simulink model "Simscape_Simulink_Mass_Spring_Damper_RL"  (R2024b)
settings: Solver=VariableStepAuto  StartTime=0.0  StopTime=10.0  RelTol=1e-3
undefined symbols (not defined in the file or in its folder): DiscIntNeverNeededParam, X, Y, Z
libraries: sm_lib x10, nesl_utility x3, simulink x1, rllib x1
settings Model: Creator=JEETKUMAR PATEL  LastModifiedBy=JEETKUMAR PATEL

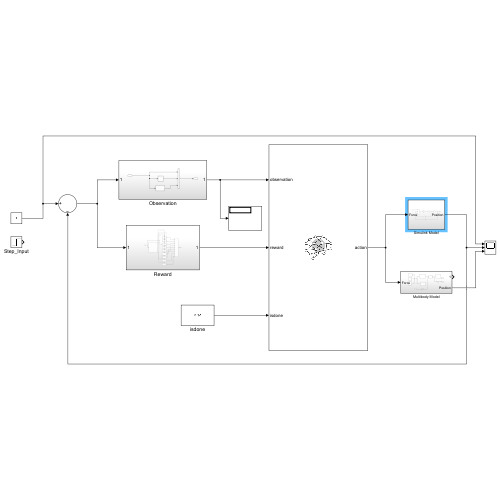
[thumbnail: Simulink's stored preview of the top-level diagram]
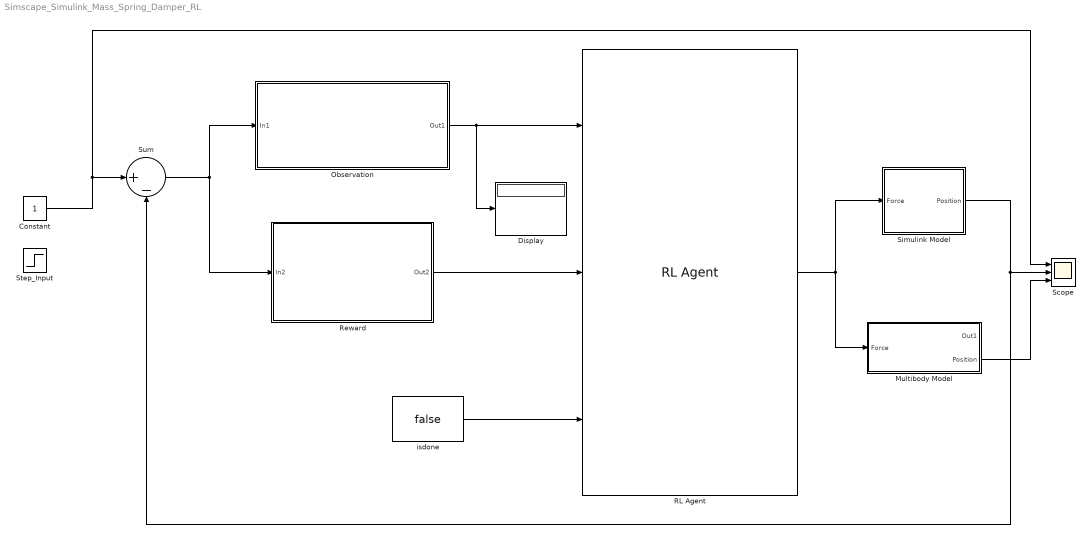
== system Simscape_Simulink_Mass_Spring_Damper_RL ==
  Constant : Constant
  Display : Display
  Multibody Model : Subsystem
  Observation : Subsystem
  RL Agent : rllib/RL Agent  Agent=agent  ExternalActionAsInput=off  ProvideLastAction=off  ProvideCumRwd=off  TreatAsDirectFeedthrough=on  UseStrictObservationDataTypes=off
  Reward : Subsystem
  Scope : Scope  NumInputPorts=3
  Simulink Model : Subsystem
  Step_Input : Step  SampleTime=0
  Sum : Sum  Inputs=|+-
  isdone : Constant  Value=false
  wires:
  Observation/1(Out1) -> RL Agent/1, Display/1
  Sum/1 -> Observation/1(In1), Reward/1(In2)
  Reward/1(Out2) -> RL Agent/2
  Constant/1 -> Sum/1, Scope/1
  Simulink Model/1(Position) -> Sum/2, Scope/2
  RL Agent/1 -> Multibody Model/1(Force), Simulink Model/1(Force)
  isdone/1 -> RL Agent/3
  Multibody Model/2(Position) -> Scope/3

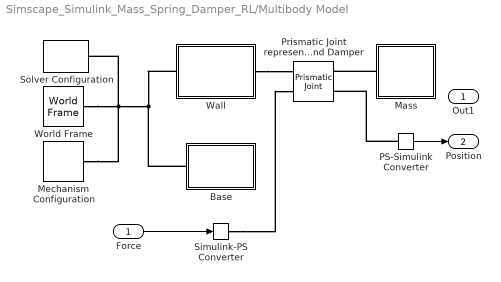
== system Simscape_Simulink_Mass_Spring_Damper_RL/Multibody Model ==
  Force : Inport
  Base : Subsystem
  Mass : Subsystem
  Mechanism Configuration : sm_lib/Utilities/Mechanism Configuration  UniformGravity=Constant  GravityVector=[0 0 -9.80665]  GravityVectorUnits=m/s^2  LinearizationDelta=0.001  JointModeTransitionNonlinearIterations=2
  PS-Simulink Converter : nesl_utility/PS-Simulink Converter  PhysicalDomain=network_engine_domain  SubClassName=ps_output  LeftPortType=input  RightPortType=output  PseudoPeriodic=off  Frequencies=[]  VectorFormat=1-D array  Unit=1  AffineConversion=off
  Prismatic Joint representing Spring and Damper : sm_lib/Joints/Prismatic Joint  JointMode=Normal  CompositeWrenchDir=FollowerOnBase  CompositeWrenchFrame=BaseFrame  SenseConstraintForce=off  SenseConstraintTorque=off  SenseTotalForce=off  SenseTotalTorque=off  PositionTargetSpecify=off  PositionTargetPriority=High  PositionTargetValue=0  PositionTargetValueUnits=m  VelocityTargetSpecify=off  VelocityTargetPriority=High  VelocityTargetValue=0  VelocityTargetValueUnits=m/s  EquilibriumPosition=0  EquilibriumPositionUnits=m  SpringStiffness=1  SpringStiffnessUnits=N/m  DampingCoefficient=1  DampingCoefficientUnits=N/(m/s)  LowerLimitSpecify=off  LowerLimitBound=-1  LowerLimitBoundUnits=m  LowerLimitStiffness=1e6  LowerLimitStiffnessUnits=N/m  LowerLimitDamping=1e3  LowerLimitDampingUnits=N/(m/s)  LowerLimitTransitionRegionWidth=1e-4  LowerLimitTransitionRegionWidthUnits=m  UpperLimitSpecify=off  UpperLimitBound=1  UpperLimitBoundUnits=m  UpperLimitStiffness=1e6  UpperLimitStiffnessUnits=N/m  UpperLimitDamping=1e3  UpperLimitDampingUnits=N/(m/s)  UpperLimitTransitionRegionWidth=1e-4  UpperLimitTransitionRegionWidthUnits=m  TorqueActuationMode=InputTorque  MotionActuationMode=ComputedMotion  SensePosition=on  SenseVelocity=off  SenseAcceleration=off  SenseTorqueForce=off  SenseLowerLimitTorqueForce=off  SenseUpperLimitTorqueForce=off
  Simulink-PS Converter : nesl_utility/Simulink-PS Converter  PhysicalDomain=network_engine_domain  SubClassName=ps_input  LeftPortType=input  RightPortType=output  PseudoPeriodic=off  Frequencies=[]  NoiseDistribution=none  NoiseParameters=[]  Unit=1  AffineConversion=off  FilteringAndDerivatives=provide  SimscapeFilterOrder=1  InputFilterTimeConstant=0.001  UdotUserProvided=0
  Solver Configuration : nesl_utility/Solver Configuration  PhysicalDomain=network_engine_domain  SubClassName=solver  LeftPortType=input  RightPortType=generic  Tones=[]  Harmonics=[]  SimulateNoise=off  Profile=off  UseLocalSampling=off  EnableSwitchedLinearOptims=on  FrequencyDomain=off  UseCCode=off  RelTol=0.001  AbsTol=1e-06  MinStep=1e-09  ToWorkspace=off  RevertToSquareIcSolve=off  NumHomotopyIterations=100  PhasorMode=off  PhasorModeNumHarmonics=1  ConsistencySolver=NEWTON_FTOL  IndexReductionMethod=DerivativeReplacement  DoDC=off  ResidualTolerance=1e-09  ConsistencyTolSource=GLOBAL  ConsistencyAbsTol=0.001  ConsistencyRelTol=0.001  ConsistencyTolFactor=0.001  UseLocalSolver=off  LocalSolverChoice=NE_BACKWARD_EULER_ADVANCER  ResolveIndetEquations=on  FunctionEvalNumThread=1  LocalSolverSampleTime=0.001  DoFixedCost=off  MaxNonlinIter=3  MaxModeIter=2  ComputeImpulses=off  ImpulseIterations=2  LinearAlgebra=auto  LinearAlgebraNumThread=0  EquationFormulation=NE_TIME_EF  DelaysMemoryBudget=1024  AutomaticFiltering=on  FilteringTimeConstant=0.001  PartitionStorageMethod=AS_NEEDED  PartitionMemoryBudget=1024  PartitionMethod=ROBUST  MultibodyUseLocalSolver=off  MultibodyLocalSolverChoice=ODE1  MultibodyLocalSolverSampleTime=0.001
  Wall : Subsystem
  World Frame : sm_lib/Frames and Transforms/World Frame
  Out1 : Outport
  Position : Outport  Port=2  VectorParamsAs1DForOutWhenUnconnected=off
  wires:
  PS-Simulink Converter/1 -> Position/1
  Force/1 -> Simulink-PS Converter/1
  connections:
  World Frame/RConn1 -- Base/LConn1 -- Wall/LConn1 -- Solver Configuration/RConn1 -- Mechanism Configuration/RConn1
  Mass/LConn1 -- Prismatic Joint representing Spring and Damper/RConn1
  Wall/RConn1 -- Prismatic Joint representing Spring and Damper/LConn1
  PS-Simulink Converter/LConn1 -- Prismatic Joint representing Spring and Damper/RConn2
  Simulink-PS Converter/RConn1 -- Prismatic Joint representing Spring and Damper/LConn2

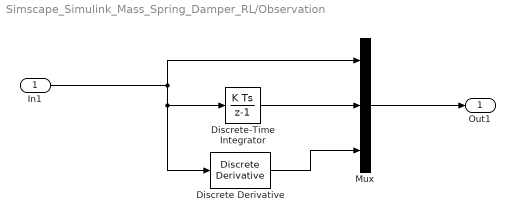
== system Simscape_Simulink_Mass_Spring_Damper_RL/Observation ==
  In1 : Inport
  Discrete Derivative : simulink/Discrete/Discrete Derivative  gainval=1.0  ICPrevScaledInput=0.0  OutMin=[]  OutMax=[]  OutDataType=fixdt(1, 16)  OutScaling=2^-10  DoSatur=off
  Discrete-Time Integrator : DiscreteIntegrator  SampleTime=-1  ICPrevOutput=DiscIntNeverNeededParam  ICPrevScaledInput=DiscIntNeverNeededParam
  Mux : Mux  Inputs=3
  Out1 : Outport
  wires:
  Discrete Derivative/1 -> Mux/3
  In1/1 -> Discrete Derivative/1, Discrete-Time Integrator/1, Mux/1
  Mux/1 -> Out1/1
  Discrete-Time Integrator/1 -> Mux/2

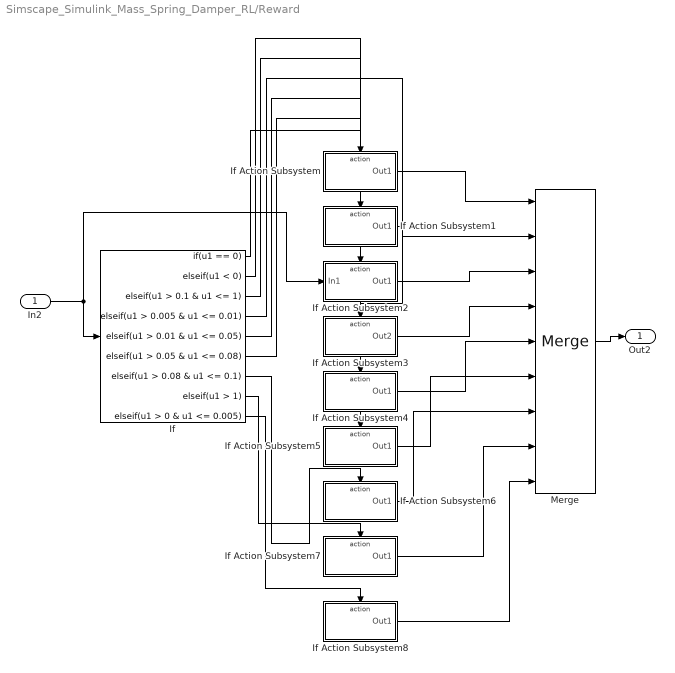
== system Simscape_Simulink_Mass_Spring_Damper_RL/Reward ==
  In2 : Inport
  If : If  IfExpression=u1 == 0  ElseIfExpressions="u1 < 0, u1 > 0.1 & u1 <= 1, u1 > 0.005 & u1 <= 0.01,  u1 > 0.01 & u1 <= 0.05, u1 > 0.05 & u1 <= 0.08, u1 > 0.08 & u1 <= 0.1, u1 > 1, u1 > 0 & u1 <= 0.005"  ShowElse=off
  If Action Subsystem : Subsystem  TreatAsAtomicUnit=on
  If Action Subsystem1 : Subsystem  TreatAsAtomicUnit=on
  If Action Subsystem2 : Subsystem  TreatAsAtomicUnit=on
  If Action Subsystem3 : Subsystem  TreatAsAtomicUnit=on
  If Action Subsystem4 : Subsystem  TreatAsAtomicUnit=on
  If Action Subsystem5 : Subsystem  TreatAsAtomicUnit=on
  If Action Subsystem6 : Subsystem  TreatAsAtomicUnit=on
  If Action Subsystem7 : Subsystem  TreatAsAtomicUnit=on
  If Action Subsystem8 : Subsystem  TreatAsAtomicUnit=on
  Merge : Merge  Inputs=9
  Out2 : Outport
  wires:
  If Action Subsystem7/1(Out1) -> Merge/8
  If Action Subsystem6/1(Out1) -> Merge/7
  If Action Subsystem/1(Out1) -> Merge/1
  If/3 -> If Action Subsystem2/Action
  If/8 -> If Action Subsystem7/Action
  If Action Subsystem2/1(Out1) -> Merge/3
  If Action Subsystem3/1(Out2) -> Merge/4
  If Action Subsystem4/1(Out1) -> Merge/5
  If Action Subsystem1/1(Out1) -> Merge/2
  If/1 -> If Action Subsystem/Action
  If/4 -> If Action Subsystem3/Action
  If/7 -> If Action Subsystem6/Action
  If/5 -> If Action Subsystem4/Action
  In2/1 -> If Action Subsystem2/1(In1), If/1
  If Action Subsystem5/1(Out1) -> Merge/6
  Merge/1 -> Out2/1
  If/6 -> If Action Subsystem5/Action
  If/2 -> If Action Subsystem1/Action
  If/9 -> If Action Subsystem8/Action
  If Action Subsystem8/1(Out1) -> Merge/9

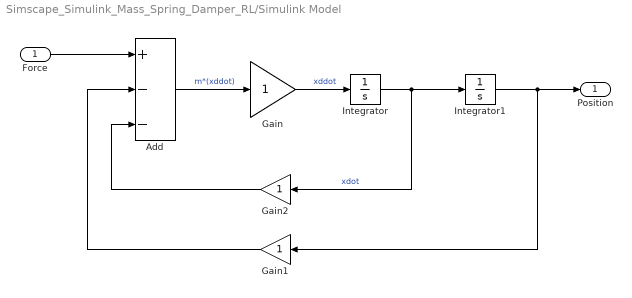
== system Simscape_Simulink_Mass_Spring_Damper_RL/Simulink Model ==
  Force : Inport
  Add : Sum  Inputs=+--
  Gain : Gain
  Gain1 : Gain
  Gain2 : Gain
  Integrator : Integrator
  Integrator1 : Integrator
  Position : Outport  VectorParamsAs1DForOutWhenUnconnected=off
  wires:
  Force/1 -> Add/1
  Add/1 -> Gain/1  "m*(xddot)"
  Integrator/1 -> Integrator1/1, Gain2/1  "xdot"
  Integrator1/1 -> Position/1, Gain1/1
  Gain1/1 -> Add/2
  Gain/1 -> Integrator/1  "xddot"
  Gain2/1 -> Add/3

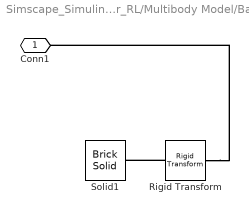
== system Simscape_Simulink_Mass_Spring_Damper_RL/Multibody Model/Base ==
  Rigid Transform : sm_lib/Frames and Transforms/Rigid Transform  RotationMethod=None  FollAlignAxisA=+X  BaseAlignAxisA=+Y  FollAlignAxisB=+Y  BaseAlignAxisB=+Z  RotationStandardAxis=+Z  RotationAngle=0.0  RotationAngleUnits=deg  RotationArbitraryAxis=[0 0 1]  RotationSequenceAxes=FollowerAxes  RotationSequence=XYX  RotationSequenceAngles=[0 0 0]  RotationSequenceAnglesUnits=deg  RotationMatrix=[1 0 0; 0 1 0; 0 0 1]  Quaternion=[1 0 0 0]  TranslationMethod=Cartesian  TranslationCartesianOffset=[1 0 -0.45]  TranslationCartesianOffsetUnits=m  TranslationStandardAxis=+Z  TranslationStandardOffset=0  TranslationStandardOffsetUnits=m  TranslationROffset=0  TranslationROffsetUnits=m  TranslationThetaOffset=0  TranslationThetaOffsetUnits=deg  TranslationZOffset=0  TranslationZOffsetUnits=m
  Solid1 : sm_lib/Body Elements/Brick Solid  BrickDimensions=[2 0.3 0.1]  BrickDimensionsUnits=m  ExportEntireGeometry=off  InertiaType=CalculateFromGeometry  BasedOnType=Density  Density=1000  DensityUnits=kg/m^3  Mass=1  MassUnits=kg  CenterOfMass=[0 0 0]  CenterOfMassUnits=m  MomentsOfInertia=[1 1 1]  MomentsOfInertiaUnits=kg*m^2  ProductsOfInertia=[0 0 0]  ProductsOfInertiaUnits=kg*m^2  GraphicType=FromGeometry  MarkerShape=Sphere  MarkerSize=10  GraphicVisPropType=SimpleVisualProperties  GraphicDiffuseColor=[0.2 0.2 1.0]  GraphicOpacity=1.0  GraphicSpecularColor=[0.5 0.5 0.5 1.0]  GraphicAmbientColor=[0.15 0.15 0.15 1.0]  GraphicEmissiveColor=[0.0 0.0 0.0 1.0]  GraphicShininess=75  DoExposeReferenceFrame=on  SerializedFrames=<Frames/>
  Conn1 : PMIOPort  Side=Left
  connections:
  Rigid Transform/RConn1 -- Solid1/RConn1
  Rigid Transform/LConn1 -- Conn1/RConn1

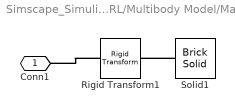
== system Simscape_Simulink_Mass_Spring_Damper_RL/Multibody Model/Mass ==
  Rigid Transform1 : sm_lib/Frames and Transforms/Rigid Transform  RotationMethod=None  FollAlignAxisA=+X  BaseAlignAxisA=+Y  FollAlignAxisB=+Y  BaseAlignAxisB=+Z  RotationStandardAxis=+Z  RotationAngle=0.0  RotationAngleUnits=deg  RotationArbitraryAxis=[0 0 1]  RotationSequenceAxes=FollowerAxes  RotationSequence=XYX  RotationSequenceAngles=[0 0 0]  RotationSequenceAnglesUnits=deg  RotationMatrix=[1 0 0; 0 1 0; 0 0 1]  Quaternion=[1 0 0 0]  TranslationMethod=Cartesian  TranslationCartesianOffset=[0 0 0.35]  TranslationCartesianOffsetUnits=m  TranslationStandardAxis=+Z  TranslationStandardOffset=0  TranslationStandardOffsetUnits=m  TranslationROffset=0  TranslationROffsetUnits=m  TranslationThetaOffset=0  TranslationThetaOffsetUnits=deg  TranslationZOffset=0  TranslationZOffsetUnits=m
  Solid1 : sm_lib/Body Elements/Brick Solid  BrickDimensions=[0.3 0.3 0.3]  BrickDimensionsUnits=m  ExportEntireGeometry=off  InertiaType=CalculateFromGeometry  BasedOnType=Mass  Density=1000  DensityUnits=kg/m^3  Mass=1  MassUnits=kg  CenterOfMass=[0 0 0]  CenterOfMassUnits=m  MomentsOfInertia=[1 1 1]  MomentsOfInertiaUnits=kg*m^2  ProductsOfInertia=[0 0 0]  ProductsOfInertiaUnits=kg*m^2  GraphicType=FromGeometry  MarkerShape=Sphere  MarkerSize=10  GraphicVisPropType=SimpleVisualProperties  GraphicDiffuseColor=[1.0 0.0 0.0]  GraphicOpacity=1.0  GraphicSpecularColor=[0.5 0.5 0.5 1.0]  GraphicAmbientColor=[0.15 0.15 0.15 1.0]  GraphicEmissiveColor=[0.0 0.0 0.0 1.0]  GraphicShininess=75  DoExposeReferenceFrame=on  SerializedFrames=<Frames/>
  Conn1 : PMIOPort  Side=Left
  connections:
  Solid1/RConn1 -- Rigid Transform1/RConn1
  Rigid Transform1/LConn1 -- Conn1/RConn1

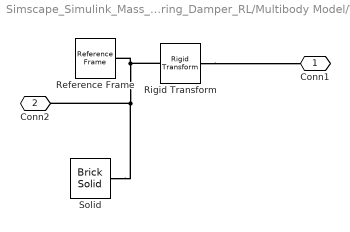
== system Simscape_Simulink_Mass_Spring_Damper_RL/Multibody Model/Wall ==
  Reference Frame : sm_lib/Frames and Transforms/Reference Frame
  Rigid Transform : sm_lib/Frames and Transforms/Rigid Transform  RotationMethod=StandardAxis  FollAlignAxisA=+X  BaseAlignAxisA=+Y  FollAlignAxisB=+Y  BaseAlignAxisB=+Z  RotationStandardAxis=+Y  RotationAngle=90  RotationAngleUnits=deg  RotationArbitraryAxis=[0 0 1]  RotationSequenceAxes=FollowerAxes  RotationSequence=XYX  RotationSequenceAngles=[0 0 0]  RotationSequenceAnglesUnits=deg  RotationMatrix=[1 0 0; 0 1 0; 0 0 1]  Quaternion=[1 0 0 0]  TranslationMethod=Cartesian  TranslationCartesianOffset=[0 0 -0.25]  TranslationCartesianOffsetUnits=m  TranslationStandardAxis=+Z  TranslationStandardOffset=0  TranslationStandardOffsetUnits=m  TranslationROffset=0  TranslationROffsetUnits=m  TranslationThetaOffset=0  TranslationThetaOffsetUnits=deg  TranslationZOffset=0  TranslationZOffsetUnits=m
  Solid : sm_lib/Body Elements/Brick Solid  BrickDimensions=[0.1 0.3 1]  BrickDimensionsUnits=m  ExportEntireGeometry=off  InertiaType=CalculateFromGeometry  BasedOnType=Density  Density=1000  DensityUnits=kg/m^3  Mass=1  MassUnits=kg  CenterOfMass=[0 0 0]  CenterOfMassUnits=m  MomentsOfInertia=[1 1 1]  MomentsOfInertiaUnits=kg*m^2  ProductsOfInertia=[0 0 0]  ProductsOfInertiaUnits=kg*m^2  GraphicType=FromGeometry  MarkerShape=Sphere  MarkerSize=10  GraphicVisPropType=SimpleVisualProperties  GraphicDiffuseColor=[0.2 0.2 1.0]  GraphicOpacity=1.0  GraphicSpecularColor=[0.5 0.5 0.5 1.0]  GraphicAmbientColor=[0.15 0.15 0.15 1.0]  GraphicEmissiveColor=[0.0 0.0 0.0 1.0]  GraphicShininess=75  DoExposeReferenceFrame=on  SerializedFrames=<Frames/>
  Conn1 : PMIOPort  Side=Right
  Conn2 : PMIOPort  Port=2  Side=Left
  connections:
  Rigid Transform/RConn1 -- Conn1/RConn1
  Rigid Transform/LConn1 -- Solid/RConn1 -- Conn2/RConn1 -- Reference Frame/RConn1

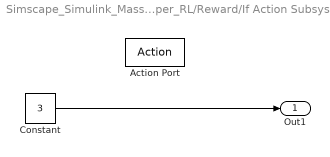
== system Simscape_Simulink_Mass_Spring_Damper_RL/Reward/If Action Subsystem ==
  Action Port : ActionPort  ActionPortLabel=if(u1 == 0)
  Constant : Constant  Value=3
  Out1 : Outport
  wires:
  Constant/1 -> Out1/1

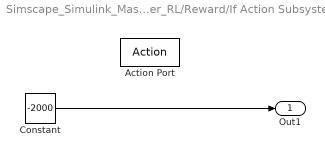
== system Simscape_Simulink_Mass_Spring_Damper_RL/Reward/If Action Subsystem1 ==
  Action Port : ActionPort  ActionPortLabel=elseif(u1 < 0)
  Constant : Constant  Value=-2000
  Out1 : Outport
  wires:
  Constant/1 -> Out1/1

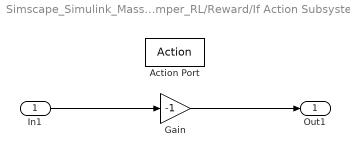
== system Simscape_Simulink_Mass_Spring_Damper_RL/Reward/If Action Subsystem2 ==
  In1 : Inport
  Action Port : ActionPort  ActionPortLabel=elseif( u1 > 0.1 & u1 <= 1)
  Gain : Gain  Gain=-1
  Out1 : Outport
  wires:
  In1/1 -> Gain/1
  Gain/1 -> Out1/1

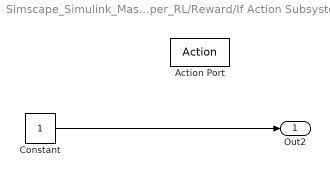
== system Simscape_Simulink_Mass_Spring_Damper_RL/Reward/If Action Subsystem3 ==
  Action Port : ActionPort  ActionPortLabel=elseif( u1 > 0.005 & u1 <= 0.01)
  Constant : Constant
  Out2 : Outport
  wires:
  Constant/1 -> Out2/1

== system Simscape_Simulink_Mass_Spring_Damper_RL/Reward/If Action Subsystem4 ==
  Action Port : ActionPort  ActionPortLabel="elseif(  u1 > 0.01 & u1 <= 0.05)"
  Constant : Constant  Value=0.4
  Out1 : Outport
  wires:
  Constant/1 -> Out1/1

== system Simscape_Simulink_Mass_Spring_Damper_RL/Reward/If Action Subsystem5 ==
  Action Port : ActionPort  ActionPortLabel=elseif( u1 > 0.05 & u1 <= 0.08)
  Constant : Constant  Value=0.2
  Out1 : Outport
  wires:
  Constant/1 -> Out1/1

== system Simscape_Simulink_Mass_Spring_Damper_RL/Reward/If Action Subsystem6 ==
  Action Port : ActionPort  ActionPortLabel=elseif( u1 > 0.08 & u1 <= 0.1)
  Constant : Constant  Value=0.1
  Out1 : Outport
  wires:
  Constant/1 -> Out1/1

== system Simscape_Simulink_Mass_Spring_Damper_RL/Reward/If Action Subsystem7 ==
  Action Port : ActionPort  ActionPortLabel=elseif( u1 > 1)
  Constant : Constant  Value=-100
  Out1 : Outport
  wires:
  Constant/1 -> Out1/1

== system Simscape_Simulink_Mass_Spring_Damper_RL/Reward/If Action Subsystem8 ==
  Action Port : ActionPort  ActionPortLabel=elseif( u1 > 0 & u1 <= 0.005)
  Constant : Constant  Value=2
  Out1 : Outport
  wires:
  Constant/1 -> Out1/1
